simulink model "hx"  (R2021a)
settings: Solver=ode1  StartTime=0.0  StopTime=120  FixedStep=0.1  RelTol=1e-3
InitFcn:
  | hx_parameters
values from neighbouring files (symbols this model uses):
  A = 380    [hx_parameters.m]
  cp1 = 4190    [hx_parameters.m]
  cp2 = 4190    [hx_parameters.m]
  h = 6800    [hx_parameters.m]
  m1 = 400    [hx_parameters.m]
  m2 = 400    [hx_parameters.m]
  T1_ini = 68    [hx_parameters.m]
  T2_ini = 91    [hx_parameters.m]
settings Model: Creator=Mikael  LastModifiedBy=Mikael

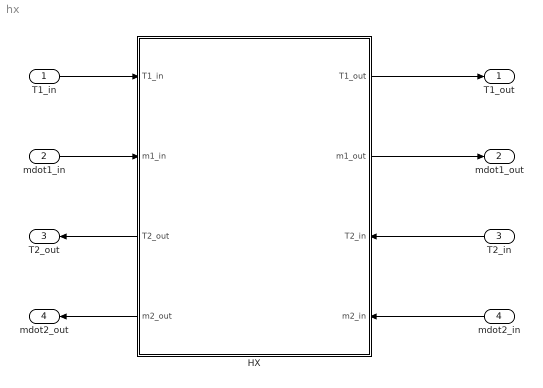
== system hx ==
  T1_in : Inport
  mdot1_in : Inport  Port=2
  T2_in : Inport  Port=3
  mdot2_in : Inport  Port=4
  HX : Subsystem
      settings: PortSchema="{\"entries\":[{\"content\":{\"sides\":[{\"content\":{\"connectorIds\":[\"In1\",\"In2\",\"Out3\",\"Out4\"]},\"type\":\"ConnectorPlacement.EquallySpacedRectSide\",\"uuid\":\"b608803e-13f5-49cd-ab3a-92503d47ac52\"},{\"content\":{\"connectorIds\":[\"Out1\",\"Out2\",\"In3\",\"In4\"],\"side\":\"RIGHT\"},\"type\":\"ConnectorPlacement.EquallySpacedRectSide\",\"uuid\":\"cb859c45-d915-447d-9a89-62abad3e0c6f\"},{\"content\":{\"connectorIds\":[],\"side\":\"TOP\"},\"type\":\"ConnectorPlacement.EquallySpacedRectSide\",\"uuid\":\"d365d95d-a075-458d-ace5-a17a7cf71809\"}]},\"type\":\"ConnectorPlacement.EquallySpacedConnector\",\"uuid\":\"ca673d01-47a6-46be-9ba4-be473b696b68\"}],\"packageUris\":[\"http://schema.mathworks.com/mf0/Connector/R2020b\"],\"version\":\"1.0\"}"
  T1_out : Outport
  mdot1_out : Outport  Port=2
  T2_out : Outport  Port=3
  mdot2_out : Outport  Port=4
  wires:
  T1_in/1 -> HX/1(T1_in)
  mdot1_in/1 -> HX/2(m1_in)
  T2_in/1 -> HX/3(T2_in)
  mdot2_in/1 -> HX/4(m2_in)
  HX/1(T1_out) -> T1_out/1
  HX/2(m1_out) -> mdot1_out/1
  HX/3(T2_out) -> T2_out/1
  HX/4(m2_out) -> mdot2_out/1

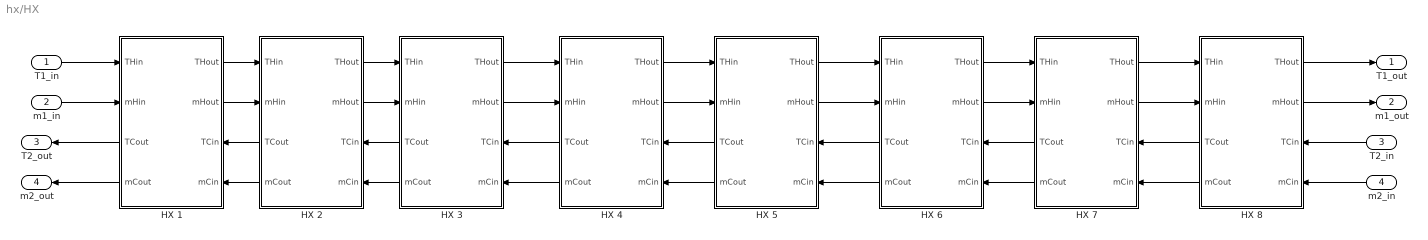
== system hx/HX ==
  T1_in : Inport
  m1_in : Inport  Port=2
  T2_in : Inport  Port=3
  m2_in : Inport  Port=4
  HX 1 : Subsystem
      settings: PortSchema="{\"entries\":[{\"content\":{\"sides\":[{\"content\":{\"connectorIds\":[\"In1\",\"In2\",\"Out3\",\"Out4\"]},\"type\":\"ConnectorPlacement.EquallySpacedRectSide\",\"uuid\":\"b608803e-13f5-49cd-ab3a-92503d47ac52\"},{\"content\":{\"connectorIds\":[\"Out1\",\"Out2\",\"In3\",\"In4\"],\"side\":\"RIGHT\"},\"type\":\"ConnectorPlacement.EquallySpacedRectSide\",\"uuid\":\"cb859c45-d915-447d-9a89-62abad3e0c6f\"},{\"content\":{\"connectorIds\":[],\"side\":\"TOP\"},\"type\":\"ConnectorPlacement.EquallySpacedRectSide\",\"uuid\":\"d365d95d-a075-458d-ace5-a17a7cf71809\"}]},\"type\":\"ConnectorPlacement.EquallySpacedConnector\",\"uuid\":\"ca673d01-47a6-46be-9ba4-be473b696b68\"}],\"packageUris\":[\"http://schema.mathworks.com/mf0/Connector/R2020b\"],\"version\":\"1.0\"}"
  HX 2 : Subsystem
      settings: PortSchema="{\"entries\":[{\"content\":{\"sides\":[{\"content\":{\"connectorIds\":[\"In1\",\"In2\",\"Out3\",\"Out4\"]},\"type\":\"ConnectorPlacement.EquallySpacedRectSide\",\"uuid\":\"b608803e-13f5-49cd-ab3a-92503d47ac52\"},{\"content\":{\"connectorIds\":[\"Out1\",\"Out2\",\"In3\",\"In4\"],\"side\":\"RIGHT\"},\"type\":\"ConnectorPlacement.EquallySpacedRectSide\",\"uuid\":\"cb859c45-d915-447d-9a89-62abad3e0c6f\"},{\"content\":{\"connectorIds\":[],\"side\":\"TOP\"},\"type\":\"ConnectorPlacement.EquallySpacedRectSide\",\"uuid\":\"d365d95d-a075-458d-ace5-a17a7cf71809\"}]},\"type\":\"ConnectorPlacement.EquallySpacedConnector\",\"uuid\":\"ca673d01-47a6-46be-9ba4-be473b696b68\"}],\"packageUris\":[\"http://schema.mathworks.com/mf0/Connector/R2020b\"],\"version\":\"1.0\"}"
  HX 3 : Subsystem
      settings: PortSchema="{\"entries\":[{\"content\":{\"sides\":[{\"content\":{\"connectorIds\":[\"In1\",\"In2\",\"Out3\",\"Out4\"]},\"type\":\"ConnectorPlacement.EquallySpacedRectSide\",\"uuid\":\"b608803e-13f5-49cd-ab3a-92503d47ac52\"},{\"content\":{\"connectorIds\":[\"Out1\",\"Out2\",\"In3\",\"In4\"],\"side\":\"RIGHT\"},\"type\":\"ConnectorPlacement.EquallySpacedRectSide\",\"uuid\":\"cb859c45-d915-447d-9a89-62abad3e0c6f\"},{\"content\":{\"connectorIds\":[],\"side\":\"TOP\"},\"type\":\"ConnectorPlacement.EquallySpacedRectSide\",\"uuid\":\"d365d95d-a075-458d-ace5-a17a7cf71809\"}]},\"type\":\"ConnectorPlacement.EquallySpacedConnector\",\"uuid\":\"ca673d01-47a6-46be-9ba4-be473b696b68\"}],\"packageUris\":[\"http://schema.mathworks.com/mf0/Connector/R2020b\"],\"version\":\"1.0\"}"
  HX 4 : Subsystem
      settings: PortSchema="{\"entries\":[{\"content\":{\"sides\":[{\"content\":{\"connectorIds\":[\"In1\",\"In2\",\"Out3\",\"Out4\"]},\"type\":\"ConnectorPlacement.EquallySpacedRectSide\",\"uuid\":\"b608803e-13f5-49cd-ab3a-92503d47ac52\"},{\"content\":{\"connectorIds\":[\"Out1\",\"Out2\",\"In3\",\"In4\"],\"side\":\"RIGHT\"},\"type\":\"ConnectorPlacement.EquallySpacedRectSide\",\"uuid\":\"cb859c45-d915-447d-9a89-62abad3e0c6f\"},{\"content\":{\"connectorIds\":[],\"side\":\"TOP\"},\"type\":\"ConnectorPlacement.EquallySpacedRectSide\",\"uuid\":\"d365d95d-a075-458d-ace5-a17a7cf71809\"}]},\"type\":\"ConnectorPlacement.EquallySpacedConnector\",\"uuid\":\"ca673d01-47a6-46be-9ba4-be473b696b68\"}],\"packageUris\":[\"http://schema.mathworks.com/mf0/Connector/R2020b\"],\"version\":\"1.0\"}"
  HX 5 : Subsystem
      settings: PortSchema="{\"entries\":[{\"content\":{\"sides\":[{\"content\":{\"connectorIds\":[\"In1\",\"In2\",\"Out3\",\"Out4\"]},\"type\":\"ConnectorPlacement.EquallySpacedRectSide\",\"uuid\":\"b608803e-13f5-49cd-ab3a-92503d47ac52\"},{\"content\":{\"connectorIds\":[\"Out1\",\"Out2\",\"In3\",\"In4\"],\"side\":\"RIGHT\"},\"type\":\"ConnectorPlacement.EquallySpacedRectSide\",\"uuid\":\"cb859c45-d915-447d-9a89-62abad3e0c6f\"},{\"content\":{\"connectorIds\":[],\"side\":\"TOP\"},\"type\":\"ConnectorPlacement.EquallySpacedRectSide\",\"uuid\":\"d365d95d-a075-458d-ace5-a17a7cf71809\"}]},\"type\":\"ConnectorPlacement.EquallySpacedConnector\",\"uuid\":\"ca673d01-47a6-46be-9ba4-be473b696b68\"}],\"packageUris\":[\"http://schema.mathworks.com/mf0/Connector/R2020b\"],\"version\":\"1.0\"}"
  HX 6 : Subsystem
      settings: PortSchema="{\"entries\":[{\"content\":{\"sides\":[{\"content\":{\"connectorIds\":[\"In1\",\"In2\",\"Out3\",\"Out4\"]},\"type\":\"ConnectorPlacement.EquallySpacedRectSide\",\"uuid\":\"b608803e-13f5-49cd-ab3a-92503d47ac52\"},{\"content\":{\"connectorIds\":[\"Out1\",\"Out2\",\"In3\",\"In4\"],\"side\":\"RIGHT\"},\"type\":\"ConnectorPlacement.EquallySpacedRectSide\",\"uuid\":\"cb859c45-d915-447d-9a89-62abad3e0c6f\"},{\"content\":{\"connectorIds\":[],\"side\":\"TOP\"},\"type\":\"ConnectorPlacement.EquallySpacedRectSide\",\"uuid\":\"d365d95d-a075-458d-ace5-a17a7cf71809\"}]},\"type\":\"ConnectorPlacement.EquallySpacedConnector\",\"uuid\":\"ca673d01-47a6-46be-9ba4-be473b696b68\"}],\"packageUris\":[\"http://schema.mathworks.com/mf0/Connector/R2020b\"],\"version\":\"1.0\"}"
  HX 7 : Subsystem
      settings: PortSchema="{\"entries\":[{\"content\":{\"sides\":[{\"content\":{\"connectorIds\":[\"In1\",\"In2\",\"Out3\",\"Out4\"]},\"type\":\"ConnectorPlacement.EquallySpacedRectSide\",\"uuid\":\"b608803e-13f5-49cd-ab3a-92503d47ac52\"},{\"content\":{\"connectorIds\":[\"Out1\",\"Out2\",\"In3\",\"In4\"],\"side\":\"RIGHT\"},\"type\":\"ConnectorPlacement.EquallySpacedRectSide\",\"uuid\":\"cb859c45-d915-447d-9a89-62abad3e0c6f\"},{\"content\":{\"connectorIds\":[],\"side\":\"TOP\"},\"type\":\"ConnectorPlacement.EquallySpacedRectSide\",\"uuid\":\"d365d95d-a075-458d-ace5-a17a7cf71809\"}]},\"type\":\"ConnectorPlacement.EquallySpacedConnector\",\"uuid\":\"ca673d01-47a6-46be-9ba4-be473b696b68\"}],\"packageUris\":[\"http://schema.mathworks.com/mf0/Connector/R2020b\"],\"version\":\"1.0\"}"
  HX 8 : Subsystem
      settings: PortSchema="{\"entries\":[{\"content\":{\"sides\":[{\"content\":{\"connectorIds\":[\"In1\",\"In2\",\"Out3\",\"Out4\"]},\"type\":\"ConnectorPlacement.EquallySpacedRectSide\",\"uuid\":\"b608803e-13f5-49cd-ab3a-92503d47ac52\"},{\"content\":{\"connectorIds\":[\"Out1\",\"Out2\",\"In3\",\"In4\"],\"side\":\"RIGHT\"},\"type\":\"ConnectorPlacement.EquallySpacedRectSide\",\"uuid\":\"cb859c45-d915-447d-9a89-62abad3e0c6f\"},{\"content\":{\"connectorIds\":[],\"side\":\"TOP\"},\"type\":\"ConnectorPlacement.EquallySpacedRectSide\",\"uuid\":\"d365d95d-a075-458d-ace5-a17a7cf71809\"}]},\"type\":\"ConnectorPlacement.EquallySpacedConnector\",\"uuid\":\"ca673d01-47a6-46be-9ba4-be473b696b68\"}],\"packageUris\":[\"http://schema.mathworks.com/mf0/Connector/R2020b\"],\"version\":\"1.0\"}"
  T1_out : Outport
  m1_out : Outport  Port=2
  T2_out : Outport  Port=3
  m2_out : Outport  Port=4
  wires:
  HX 2/3(TCout) -> HX 1/3(TCin)
  HX 4/1(THout) -> HX 5/1(THin)
  HX 4/2(mHout) -> HX 5/2(mHin)
  HX 1/1(THout) -> HX 2/1(THin)
  HX 5/3(TCout) -> HX 4/3(TCin)
  m1_in/1 -> HX 1/2(mHin)
  HX 2/1(THout) -> HX 3/1(THin)
  HX 1/2(mHout) -> HX 2/2(mHin)
  HX 5/4(mCout) -> HX 4/4(mCin)
  HX 2/4(mCout) -> HX 1/4(mCin)
  HX 5/2(mHout) -> HX 6/2(mHin)
  HX 7/4(mCout) -> HX 6/4(mCin)
  HX 7/3(TCout) -> HX 6/3(TCin)
  HX 3/2(mHout) -> HX 4/2(mHin)
  HX 6/2(mHout) -> HX 7/2(mHin)
  HX 8/2(mHout) -> m1_out/1
  HX 6/1(THout) -> HX 7/1(THin)
  HX 2/2(mHout) -> HX 3/2(mHin)
  HX 3/4(mCout) -> HX 2/4(mCin)
  T2_in/1 -> HX 8/3(TCin)
  HX 3/3(TCout) -> HX 2/3(TCin)
  T1_in/1 -> HX 1/1(THin)
  HX 5/1(THout) -> HX 6/1(THin)
  HX 3/1(THout) -> HX 4/1(THin)
  HX 4/3(TCout) -> HX 3/3(TCin)
  HX 6/3(TCout) -> HX 5/3(TCin)
  HX 4/4(mCout) -> HX 3/4(mCin)
  HX 7/1(THout) -> HX 8/1(THin)
  HX 8/3(TCout) -> HX 7/3(TCin)
  HX 7/2(mHout) -> HX 8/2(mHin)
  HX 8/4(mCout) -> HX 7/4(mCin)
  HX 1/3(TCout) -> T2_out/1
  HX 6/4(mCout) -> HX 5/4(mCin)
  HX 8/1(THout) -> T1_out/1
  m2_in/1 -> HX 8/4(mCin)
  HX 1/4(mCout) -> m2_out/1

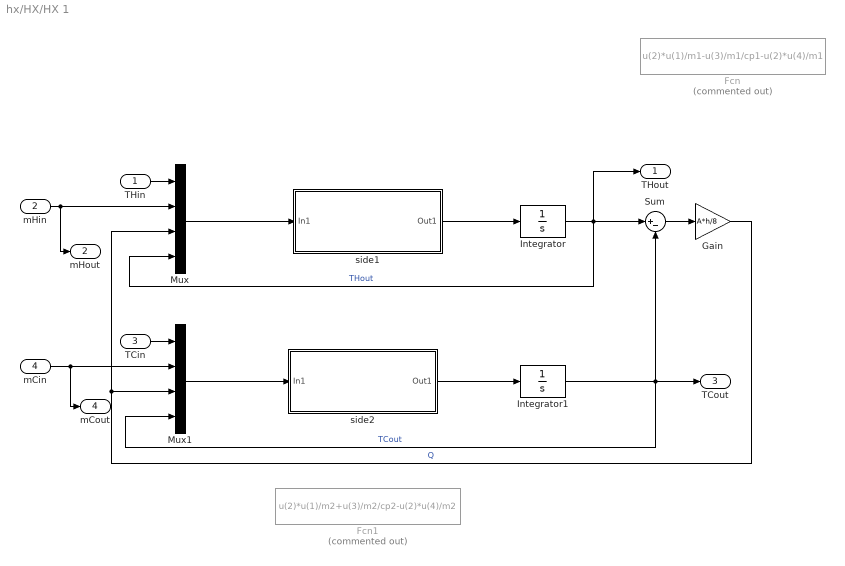
== system hx/HX/HX 1 ==
  THin : Inport
  mHin : Inport  Port=2
  TCin : Inport  Port=3
  mCin : Inport  Port=4
  Fcn : Fcn  Commented=on  Expr=u(2)*u(1)/m1-u(3)/m1/cp1-u(2)*u(4)/m1
  Fcn1 : Fcn  Commented=on  Expr=u(2)*u(1)/m2+u(3)/m2/cp2-u(2)*u(4)/m2
  Gain : Gain  Gain=A*h/8
  Integrator : Integrator  InitialCondition=T1_ini
  Integrator1 : Integrator  InitialCondition=T2_ini
  Mux : Mux
  Mux1 : Mux
  Sum : Sum  Inputs=|+-
  side1 : Subsystem
  side2 : Subsystem
  THout : Outport  VectorParamsAs1DForOutWhenUnconnected=off
  mHout : Outport  Port=2  VectorParamsAs1DForOutWhenUnconnected=off
  TCout : Outport  Port=3  VectorParamsAs1DForOutWhenUnconnected=off
  mCout : Outport  Port=4  VectorParamsAs1DForOutWhenUnconnected=off
  wires:
  Integrator/1 -> THout/1, Sum/1, Mux/4  "THout"
  Sum/1 -> Gain/1
  Mux1/1 -> side2/1(In1)
  side2/1(Out1) -> Integrator1/1
  Integrator1/1 -> Sum/2, TCout/1, Mux1/4  "TCout"
  mCin/1 -> Mux1/2, mCout/1
  TCin/1 -> Mux1/1
  THin/1 -> Mux/1
  Gain/1 -> Mux1/3, Mux/3  "Q"
  mHin/1 -> Mux/2, mHout/1
  Mux/1 -> side1/1(In1)
  side1/1(Out1) -> Integrator/1

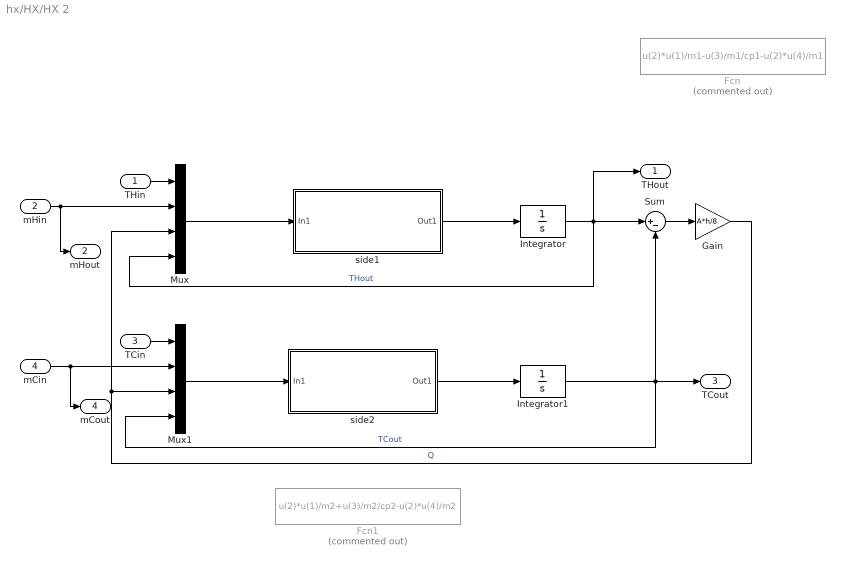
== system hx/HX/HX 2 ==
  THin : Inport
  mHin : Inport  Port=2
  TCin : Inport  Port=3
  mCin : Inport  Port=4
  Fcn : Fcn  Commented=on  Expr=u(2)*u(1)/m1-u(3)/m1/cp1-u(2)*u(4)/m1
  Fcn1 : Fcn  Commented=on  Expr=u(2)*u(1)/m2+u(3)/m2/cp2-u(2)*u(4)/m2
  Gain : Gain  Gain=A*h/8
  Integrator : Integrator  InitialCondition=T1_ini
  Integrator1 : Integrator  InitialCondition=T2_ini
  Mux : Mux
  Mux1 : Mux
  Sum : Sum  Inputs=|+-
  side1 : Subsystem
  side2 : Subsystem
  THout : Outport  VectorParamsAs1DForOutWhenUnconnected=off
  mHout : Outport  Port=2  VectorParamsAs1DForOutWhenUnconnected=off
  TCout : Outport  Port=3  VectorParamsAs1DForOutWhenUnconnected=off
  mCout : Outport  Port=4  VectorParamsAs1DForOutWhenUnconnected=off
  wires:
  side1/1(Out1) -> Integrator/1
  Mux/1 -> side1/1(In1)
  mHin/1 -> mHout/1, Mux/2
  Gain/1 -> Mux/3, Mux1/3  "Q"
  THin/1 -> Mux/1
  TCin/1 -> Mux1/1
  mCin/1 -> mCout/1, Mux1/2
  Integrator1/1 -> Mux1/4, TCout/1, Sum/2  "TCout"
  side2/1(Out1) -> Integrator1/1
  Mux1/1 -> side2/1(In1)
  Sum/1 -> Gain/1
  Integrator/1 -> Mux/4, Sum/1, THout/1  "THout"

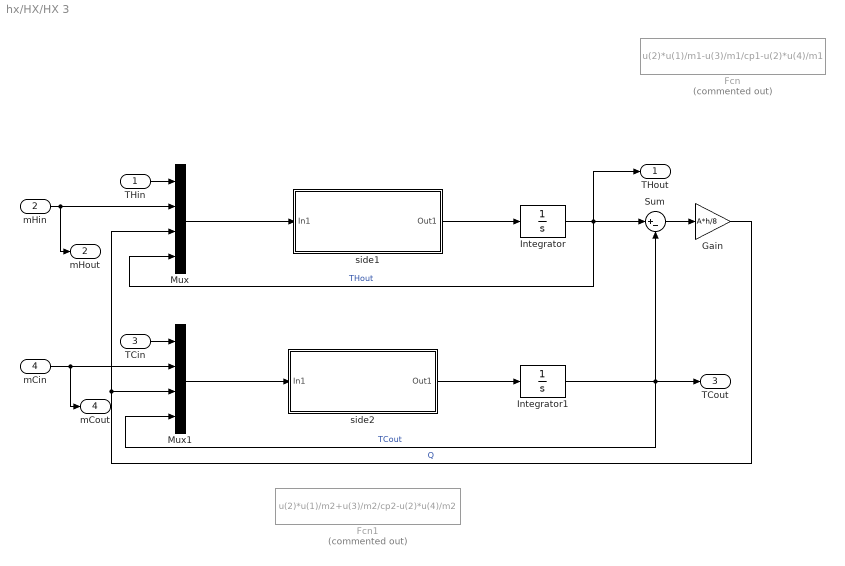
== system hx/HX/HX 3 ==
  THin : Inport
  mHin : Inport  Port=2
  TCin : Inport  Port=3
  mCin : Inport  Port=4
  Fcn : Fcn  Commented=on  Expr=u(2)*u(1)/m1-u(3)/m1/cp1-u(2)*u(4)/m1
  Fcn1 : Fcn  Commented=on  Expr=u(2)*u(1)/m2+u(3)/m2/cp2-u(2)*u(4)/m2
  Gain : Gain  Gain=A*h/8
  Integrator : Integrator  InitialCondition=T1_ini
  Integrator1 : Integrator  InitialCondition=T2_ini
  Mux : Mux
  Mux1 : Mux
  Sum : Sum  Inputs=|+-
  side1 : Subsystem
  side2 : Subsystem
  THout : Outport  VectorParamsAs1DForOutWhenUnconnected=off
  mHout : Outport  Port=2  VectorParamsAs1DForOutWhenUnconnected=off
  TCout : Outport  Port=3  VectorParamsAs1DForOutWhenUnconnected=off
  mCout : Outport  Port=4  VectorParamsAs1DForOutWhenUnconnected=off
  wires:
  Integrator/1 -> THout/1, Sum/1, Mux/4  "THout"
  Sum/1 -> Gain/1
  Mux1/1 -> side2/1(In1)
  side2/1(Out1) -> Integrator1/1
  Integrator1/1 -> Sum/2, TCout/1, Mux1/4  "TCout"
  mCin/1 -> Mux1/2, mCout/1
  TCin/1 -> Mux1/1
  THin/1 -> Mux/1
  Gain/1 -> Mux1/3, Mux/3  "Q"
  mHin/1 -> Mux/2, mHout/1
  Mux/1 -> side1/1(In1)
  side1/1(Out1) -> Integrator/1

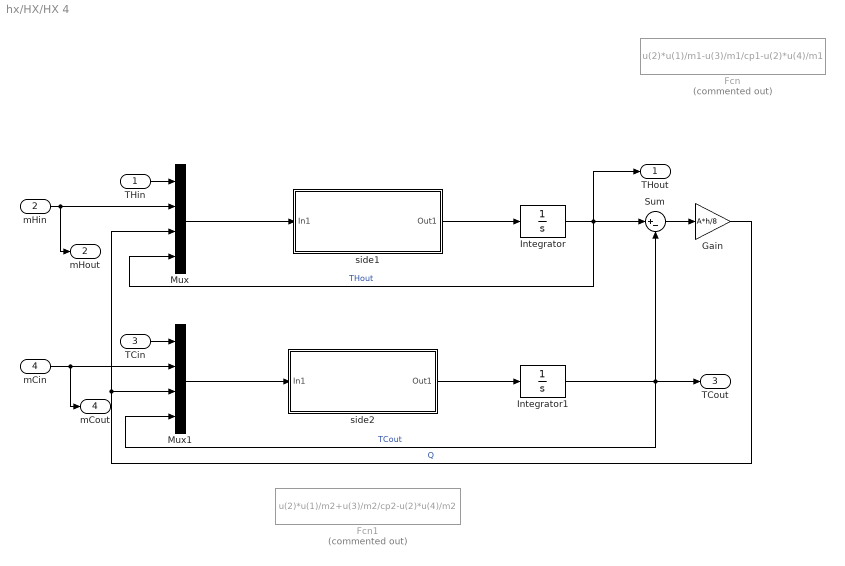
== system hx/HX/HX 4 ==
  THin : Inport
  mHin : Inport  Port=2
  TCin : Inport  Port=3
  mCin : Inport  Port=4
  Fcn : Fcn  Commented=on  Expr=u(2)*u(1)/m1-u(3)/m1/cp1-u(2)*u(4)/m1
  Fcn1 : Fcn  Commented=on  Expr=u(2)*u(1)/m2+u(3)/m2/cp2-u(2)*u(4)/m2
  Gain : Gain  Gain=A*h/8
  Integrator : Integrator  InitialCondition=T1_ini
  Integrator1 : Integrator  InitialCondition=T2_ini
  Mux : Mux
  Mux1 : Mux
  Sum : Sum  Inputs=|+-
  side1 : Subsystem
  side2 : Subsystem
  THout : Outport  VectorParamsAs1DForOutWhenUnconnected=off
  mHout : Outport  Port=2  VectorParamsAs1DForOutWhenUnconnected=off
  TCout : Outport  Port=3  VectorParamsAs1DForOutWhenUnconnected=off
  mCout : Outport  Port=4  VectorParamsAs1DForOutWhenUnconnected=off
  wires:
  side1/1(Out1) -> Integrator/1
  Mux/1 -> side1/1(In1)
  mHin/1 -> mHout/1, Mux/2
  Gain/1 -> Mux/3, Mux1/3  "Q"
  THin/1 -> Mux/1
  TCin/1 -> Mux1/1
  mCin/1 -> mCout/1, Mux1/2
  Integrator1/1 -> Mux1/4, TCout/1, Sum/2  "TCout"
  side2/1(Out1) -> Integrator1/1
  Mux1/1 -> side2/1(In1)
  Sum/1 -> Gain/1
  Integrator/1 -> Mux/4, Sum/1, THout/1  "THout"

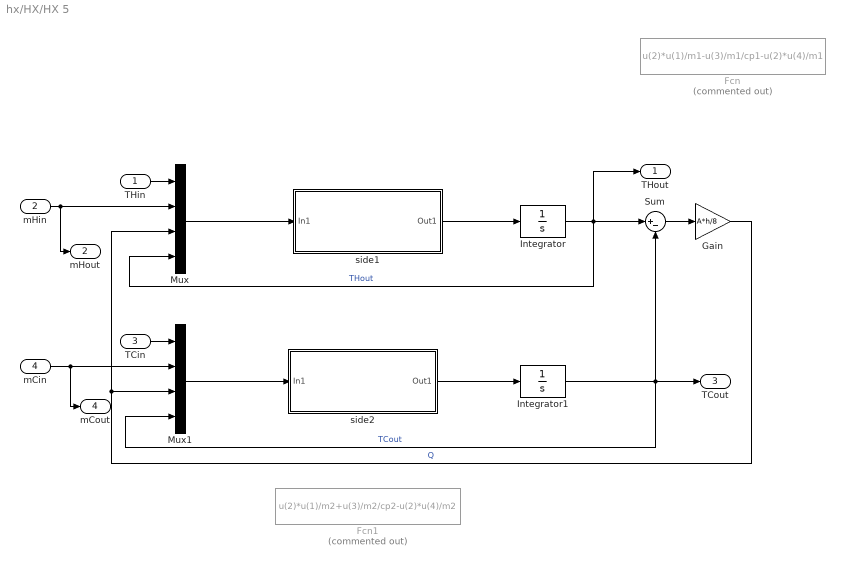
== system hx/HX/HX 5 ==
  THin : Inport
  mHin : Inport  Port=2
  TCin : Inport  Port=3
  mCin : Inport  Port=4
  Fcn : Fcn  Commented=on  Expr=u(2)*u(1)/m1-u(3)/m1/cp1-u(2)*u(4)/m1
  Fcn1 : Fcn  Commented=on  Expr=u(2)*u(1)/m2+u(3)/m2/cp2-u(2)*u(4)/m2
  Gain : Gain  Gain=A*h/8
  Integrator : Integrator  InitialCondition=T1_ini
  Integrator1 : Integrator  InitialCondition=T2_ini
  Mux : Mux
  Mux1 : Mux
  Sum : Sum  Inputs=|+-
  side1 : Subsystem
  side2 : Subsystem
  THout : Outport  VectorParamsAs1DForOutWhenUnconnected=off
  mHout : Outport  Port=2  VectorParamsAs1DForOutWhenUnconnected=off
  TCout : Outport  Port=3  VectorParamsAs1DForOutWhenUnconnected=off
  mCout : Outport  Port=4  VectorParamsAs1DForOutWhenUnconnected=off
  wires:
  Integrator/1 -> THout/1, Sum/1, Mux/4  "THout"
  Sum/1 -> Gain/1
  Mux1/1 -> side2/1(In1)
  side2/1(Out1) -> Integrator1/1
  Integrator1/1 -> Sum/2, TCout/1, Mux1/4  "TCout"
  mCin/1 -> Mux1/2, mCout/1
  TCin/1 -> Mux1/1
  THin/1 -> Mux/1
  Gain/1 -> Mux1/3, Mux/3  "Q"
  mHin/1 -> Mux/2, mHout/1
  Mux/1 -> side1/1(In1)
  side1/1(Out1) -> Integrator/1

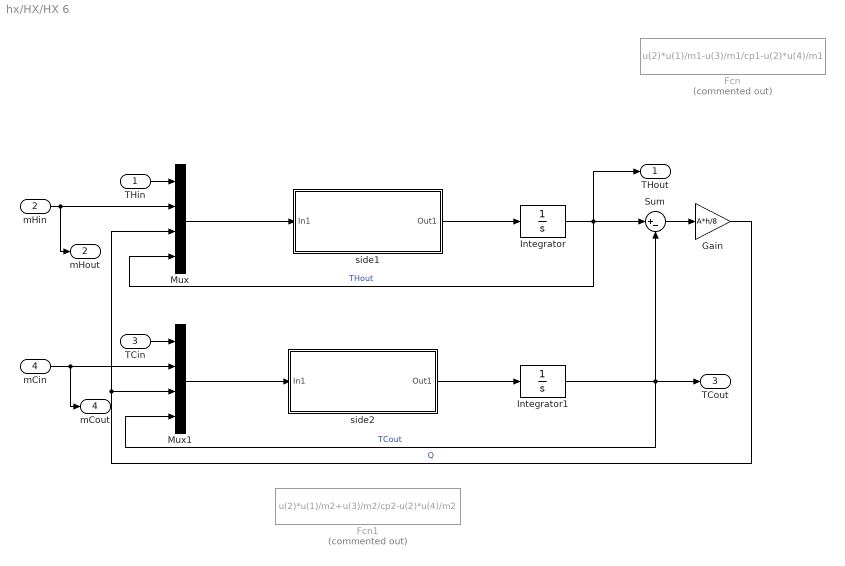
== system hx/HX/HX 6 ==
  THin : Inport
  mHin : Inport  Port=2
  TCin : Inport  Port=3
  mCin : Inport  Port=4
  Fcn : Fcn  Commented=on  Expr=u(2)*u(1)/m1-u(3)/m1/cp1-u(2)*u(4)/m1
  Fcn1 : Fcn  Commented=on  Expr=u(2)*u(1)/m2+u(3)/m2/cp2-u(2)*u(4)/m2
  Gain : Gain  Gain=A*h/8
  Integrator : Integrator  InitialCondition=T1_ini
  Integrator1 : Integrator  InitialCondition=T2_ini
  Mux : Mux
  Mux1 : Mux
  Sum : Sum  Inputs=|+-
  side1 : Subsystem
  side2 : Subsystem
  THout : Outport  VectorParamsAs1DForOutWhenUnconnected=off
  mHout : Outport  Port=2  VectorParamsAs1DForOutWhenUnconnected=off
  TCout : Outport  Port=3  VectorParamsAs1DForOutWhenUnconnected=off
  mCout : Outport  Port=4  VectorParamsAs1DForOutWhenUnconnected=off
  wires:
  side1/1(Out1) -> Integrator/1
  Mux/1 -> side1/1(In1)
  mHin/1 -> mHout/1, Mux/2
  Gain/1 -> Mux/3, Mux1/3  "Q"
  THin/1 -> Mux/1
  TCin/1 -> Mux1/1
  mCin/1 -> mCout/1, Mux1/2
  Integrator1/1 -> Mux1/4, TCout/1, Sum/2  "TCout"
  side2/1(Out1) -> Integrator1/1
  Mux1/1 -> side2/1(In1)
  Sum/1 -> Gain/1
  Integrator/1 -> Mux/4, Sum/1, THout/1  "THout"

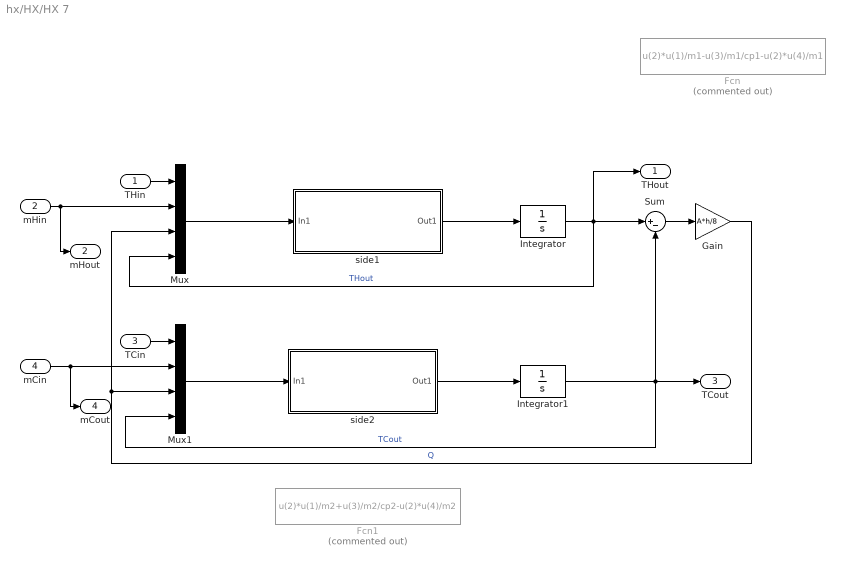
== system hx/HX/HX 7 ==
  THin : Inport
  mHin : Inport  Port=2
  TCin : Inport  Port=3
  mCin : Inport  Port=4
  Fcn : Fcn  Commented=on  Expr=u(2)*u(1)/m1-u(3)/m1/cp1-u(2)*u(4)/m1
  Fcn1 : Fcn  Commented=on  Expr=u(2)*u(1)/m2+u(3)/m2/cp2-u(2)*u(4)/m2
  Gain : Gain  Gain=A*h/8
  Integrator : Integrator  InitialCondition=T1_ini
  Integrator1 : Integrator  InitialCondition=T2_ini
  Mux : Mux
  Mux1 : Mux
  Sum : Sum  Inputs=|+-
  side1 : Subsystem
  side2 : Subsystem
  THout : Outport  VectorParamsAs1DForOutWhenUnconnected=off
  mHout : Outport  Port=2  VectorParamsAs1DForOutWhenUnconnected=off
  TCout : Outport  Port=3  VectorParamsAs1DForOutWhenUnconnected=off
  mCout : Outport  Port=4  VectorParamsAs1DForOutWhenUnconnected=off
  wires:
  Integrator/1 -> THout/1, Sum/1, Mux/4  "THout"
  Sum/1 -> Gain/1
  Mux1/1 -> side2/1(In1)
  side2/1(Out1) -> Integrator1/1
  Integrator1/1 -> Sum/2, TCout/1, Mux1/4  "TCout"
  mCin/1 -> Mux1/2, mCout/1
  TCin/1 -> Mux1/1
  THin/1 -> Mux/1
  Gain/1 -> Mux1/3, Mux/3  "Q"
  mHin/1 -> Mux/2, mHout/1
  Mux/1 -> side1/1(In1)
  side1/1(Out1) -> Integrator/1

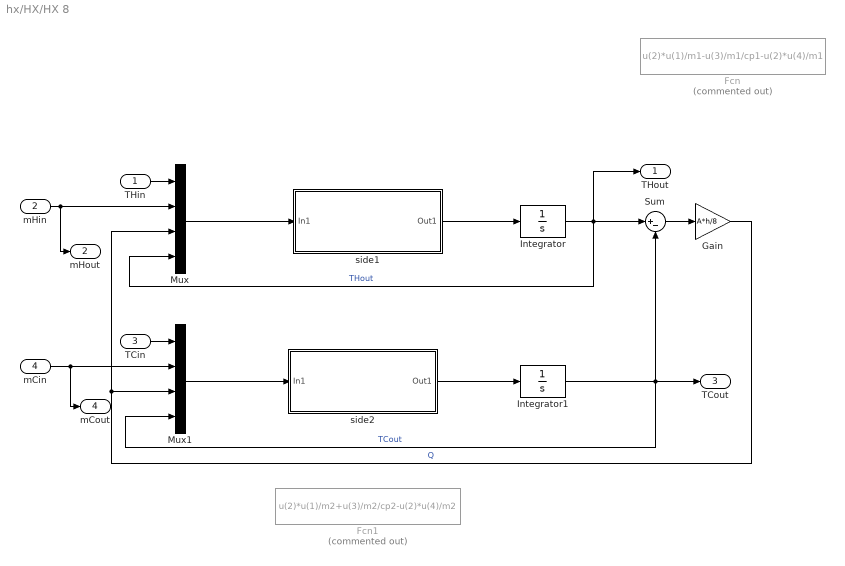
== system hx/HX/HX 8 ==
  THin : Inport
  mHin : Inport  Port=2
  TCin : Inport  Port=3
  mCin : Inport  Port=4
  Fcn : Fcn  Commented=on  Expr=u(2)*u(1)/m1-u(3)/m1/cp1-u(2)*u(4)/m1
  Fcn1 : Fcn  Commented=on  Expr=u(2)*u(1)/m2+u(3)/m2/cp2-u(2)*u(4)/m2
  Gain : Gain  Gain=A*h/8
  Integrator : Integrator  InitialCondition=T1_ini
  Integrator1 : Integrator  InitialCondition=T2_ini
  Mux : Mux
  Mux1 : Mux
  Sum : Sum  Inputs=|+-
  side1 : Subsystem
  side2 : Subsystem
  THout : Outport  VectorParamsAs1DForOutWhenUnconnected=off
  mHout : Outport  Port=2  VectorParamsAs1DForOutWhenUnconnected=off
  TCout : Outport  Port=3  VectorParamsAs1DForOutWhenUnconnected=off
  mCout : Outport  Port=4  VectorParamsAs1DForOutWhenUnconnected=off
  wires:
  side1/1(Out1) -> Integrator/1
  Mux/1 -> side1/1(In1)
  mHin/1 -> mHout/1, Mux/2
  Gain/1 -> Mux/3, Mux1/3  "Q"
  THin/1 -> Mux/1
  TCin/1 -> Mux1/1
  mCin/1 -> mCout/1, Mux1/2
  Integrator1/1 -> Mux1/4, TCout/1, Sum/2  "TCout"
  side2/1(Out1) -> Integrator1/1
  Mux1/1 -> side2/1(In1)
  Sum/1 -> Gain/1
  Integrator/1 -> Mux/4, Sum/1, THout/1  "THout"

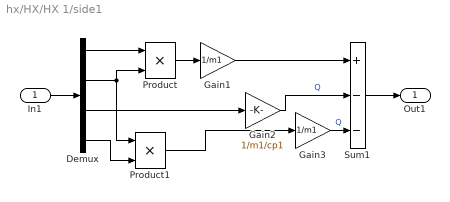
== system hx/HX/HX 1/side1 ==
  In1 : Inport
  Demux : Demux
  Gain1 : Gain  Gain=1/m1
  Gain2 : Gain  Gain=1/m1/cp1
  Gain3 : Gain  Gain=1/m1
  Product : Product
  Product1 : Product
  Sum1 : Sum  Inputs=+--
  Out1 : Outport
  wires:
  Demux/4 -> Product1/2
  Demux/3 -> Gain2/1
  Product1/1 -> Gain3/1
  Gain2/1 -> Sum1/2  "Q"
  Demux/2 -> Product/2, Product1/1
  Demux/1 -> Product/1
  Gain3/1 -> Sum1/3  "Q"
  Product/1 -> Gain1/1
  Gain1/1 -> Sum1/1
  Sum1/1 -> Out1/1
  In1/1 -> Demux/1

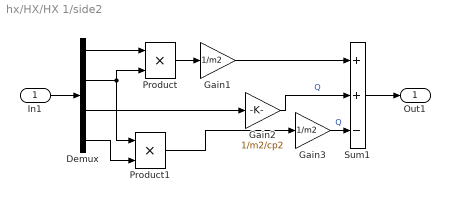
== system hx/HX/HX 1/side2 ==
  In1 : Inport
  Demux : Demux
  Gain1 : Gain  Gain=1/m2
  Gain2 : Gain  Gain=1/m2/cp2
  Gain3 : Gain  Gain=1/m2
  Product : Product
  Product1 : Product
  Sum1 : Sum  Inputs=++-
  Out1 : Outport
  wires:
  In1/1 -> Demux/1
  Sum1/1 -> Out1/1
  Gain1/1 -> Sum1/1
  Product/1 -> Gain1/1
  Gain3/1 -> Sum1/3  "Q"
  Demux/1 -> Product/1
  Demux/2 -> Product1/1, Product/2
  Gain2/1 -> Sum1/2  "Q"
  Product1/1 -> Gain3/1
  Demux/3 -> Gain2/1
  Demux/4 -> Product1/2

== system hx/HX/HX 2/side1 ==
  In1 : Inport
  Demux : Demux
  Gain1 : Gain  Gain=1/m1
  Gain2 : Gain  Gain=1/m1/cp1
  Gain3 : Gain  Gain=1/m1
  Product : Product
  Product1 : Product
  Sum1 : Sum  Inputs=+--
  Out1 : Outport
  wires:
  In1/1 -> Demux/1
  Sum1/1 -> Out1/1
  Gain1/1 -> Sum1/1
  Product/1 -> Gain1/1
  Gain3/1 -> Sum1/3  "Q"
  Demux/1 -> Product/1
  Demux/2 -> Product1/1, Product/2
  Gain2/1 -> Sum1/2  "Q"
  Product1/1 -> Gain3/1
  Demux/3 -> Gain2/1
  Demux/4 -> Product1/2

== system hx/HX/HX 2/side2 ==
  In1 : Inport
  Demux : Demux
  Gain1 : Gain  Gain=1/m2
  Gain2 : Gain  Gain=1/m2/cp2
  Gain3 : Gain  Gain=1/m2
  Product : Product
  Product1 : Product
  Sum1 : Sum  Inputs=++-
  Out1 : Outport
  wires:
  Demux/4 -> Product1/2
  Demux/3 -> Gain2/1
  Product1/1 -> Gain3/1
  Gain2/1 -> Sum1/2  "Q"
  Demux/2 -> Product/2, Product1/1
  Demux/1 -> Product/1
  Gain3/1 -> Sum1/3  "Q"
  Product/1 -> Gain1/1
  Gain1/1 -> Sum1/1
  Sum1/1 -> Out1/1
  In1/1 -> Demux/1

== system hx/HX/HX 3/side1 ==
  In1 : Inport
  Demux : Demux
  Gain1 : Gain  Gain=1/m1
  Gain2 : Gain  Gain=1/m1/cp1
  Gain3 : Gain  Gain=1/m1
  Product : Product
  Product1 : Product
  Sum1 : Sum  Inputs=+--
  Out1 : Outport
  wires:
  Demux/4 -> Product1/2
  Demux/3 -> Gain2/1
  Product1/1 -> Gain3/1
  Gain2/1 -> Sum1/2  "Q"
  Demux/2 -> Product/2, Product1/1
  Demux/1 -> Product/1
  Gain3/1 -> Sum1/3  "Q"
  Product/1 -> Gain1/1
  Gain1/1 -> Sum1/1
  Sum1/1 -> Out1/1
  In1/1 -> Demux/1

== system hx/HX/HX 3/side2 ==
  In1 : Inport
  Demux : Demux
  Gain1 : Gain  Gain=1/m2
  Gain2 : Gain  Gain=1/m2/cp2
  Gain3 : Gain  Gain=1/m2
  Product : Product
  Product1 : Product
  Sum1 : Sum  Inputs=++-
  Out1 : Outport
  wires:
  In1/1 -> Demux/1
  Sum1/1 -> Out1/1
  Gain1/1 -> Sum1/1
  Product/1 -> Gain1/1
  Gain3/1 -> Sum1/3  "Q"
  Demux/1 -> Product/1
  Demux/2 -> Product1/1, Product/2
  Gain2/1 -> Sum1/2  "Q"
  Product1/1 -> Gain3/1
  Demux/3 -> Gain2/1
  Demux/4 -> Product1/2

== system hx/HX/HX 4/side1 ==
  In1 : Inport
  Demux : Demux
  Gain1 : Gain  Gain=1/m1
  Gain2 : Gain  Gain=1/m1/cp1
  Gain3 : Gain  Gain=1/m1
  Product : Product
  Product1 : Product
  Sum1 : Sum  Inputs=+--
  Out1 : Outport
  wires:
  In1/1 -> Demux/1
  Sum1/1 -> Out1/1
  Gain1/1 -> Sum1/1
  Product/1 -> Gain1/1
  Gain3/1 -> Sum1/3  "Q"
  Demux/1 -> Product/1
  Demux/2 -> Product1/1, Product/2
  Gain2/1 -> Sum1/2  "Q"
  Product1/1 -> Gain3/1
  Demux/3 -> Gain2/1
  Demux/4 -> Product1/2

== system hx/HX/HX 4/side2 ==
  In1 : Inport
  Demux : Demux
  Gain1 : Gain  Gain=1/m2
  Gain2 : Gain  Gain=1/m2/cp2
  Gain3 : Gain  Gain=1/m2
  Product : Product
  Product1 : Product
  Sum1 : Sum  Inputs=++-
  Out1 : Outport
  wires:
  Demux/4 -> Product1/2
  Demux/3 -> Gain2/1
  Product1/1 -> Gain3/1
  Gain2/1 -> Sum1/2  "Q"
  Demux/2 -> Product/2, Product1/1
  Demux/1 -> Product/1
  Gain3/1 -> Sum1/3  "Q"
  Product/1 -> Gain1/1
  Gain1/1 -> Sum1/1
  Sum1/1 -> Out1/1
  In1/1 -> Demux/1

== system hx/HX/HX 5/side1 ==
  In1 : Inport
  Demux : Demux
  Gain1 : Gain  Gain=1/m1
  Gain2 : Gain  Gain=1/m1/cp1
  Gain3 : Gain  Gain=1/m1
  Product : Product
  Product1 : Product
  Sum1 : Sum  Inputs=+--
  Out1 : Outport
  wires:
  Demux/4 -> Product1/2
  Demux/3 -> Gain2/1
  Product1/1 -> Gain3/1
  Gain2/1 -> Sum1/2  "Q"
  Demux/2 -> Product/2, Product1/1
  Demux/1 -> Product/1
  Gain3/1 -> Sum1/3  "Q"
  Product/1 -> Gain1/1
  Gain1/1 -> Sum1/1
  Sum1/1 -> Out1/1
  In1/1 -> Demux/1

== system hx/HX/HX 5/side2 ==
  In1 : Inport
  Demux : Demux
  Gain1 : Gain  Gain=1/m2
  Gain2 : Gain  Gain=1/m2/cp2
  Gain3 : Gain  Gain=1/m2
  Product : Product
  Product1 : Product
  Sum1 : Sum  Inputs=++-
  Out1 : Outport
  wires:
  In1/1 -> Demux/1
  Sum1/1 -> Out1/1
  Gain1/1 -> Sum1/1
  Product/1 -> Gain1/1
  Gain3/1 -> Sum1/3  "Q"
  Demux/1 -> Product/1
  Demux/2 -> Product1/1, Product/2
  Gain2/1 -> Sum1/2  "Q"
  Product1/1 -> Gain3/1
  Demux/3 -> Gain2/1
  Demux/4 -> Product1/2

== system hx/HX/HX 6/side1 ==
  In1 : Inport
  Demux : Demux
  Gain1 : Gain  Gain=1/m1
  Gain2 : Gain  Gain=1/m1/cp1
  Gain3 : Gain  Gain=1/m1
  Product : Product
  Product1 : Product
  Sum1 : Sum  Inputs=+--
  Out1 : Outport
  wires:
  In1/1 -> Demux/1
  Sum1/1 -> Out1/1
  Gain1/1 -> Sum1/1
  Product/1 -> Gain1/1
  Gain3/1 -> Sum1/3  "Q"
  Demux/1 -> Product/1
  Demux/2 -> Product1/1, Product/2
  Gain2/1 -> Sum1/2  "Q"
  Product1/1 -> Gain3/1
  Demux/3 -> Gain2/1
  Demux/4 -> Product1/2

== system hx/HX/HX 6/side2 ==
  In1 : Inport
  Demux : Demux
  Gain1 : Gain  Gain=1/m2
  Gain2 : Gain  Gain=1/m2/cp2
  Gain3 : Gain  Gain=1/m2
  Product : Product
  Product1 : Product
  Sum1 : Sum  Inputs=++-
  Out1 : Outport
  wires:
  Demux/4 -> Product1/2
  Demux/3 -> Gain2/1
  Product1/1 -> Gain3/1
  Gain2/1 -> Sum1/2  "Q"
  Demux/2 -> Product/2, Product1/1
  Demux/1 -> Product/1
  Gain3/1 -> Sum1/3  "Q"
  Product/1 -> Gain1/1
  Gain1/1 -> Sum1/1
  Sum1/1 -> Out1/1
  In1/1 -> Demux/1

== system hx/HX/HX 7/side1 ==
  In1 : Inport
  Demux : Demux
  Gain1 : Gain  Gain=1/m1
  Gain2 : Gain  Gain=1/m1/cp1
  Gain3 : Gain  Gain=1/m1
  Product : Product
  Product1 : Product
  Sum1 : Sum  Inputs=+--
  Out1 : Outport
  wires:
  Demux/4 -> Product1/2
  Demux/3 -> Gain2/1
  Product1/1 -> Gain3/1
  Gain2/1 -> Sum1/2  "Q"
  Demux/2 -> Product/2, Product1/1
  Demux/1 -> Product/1
  Gain3/1 -> Sum1/3  "Q"
  Product/1 -> Gain1/1
  Gain1/1 -> Sum1/1
  Sum1/1 -> Out1/1
  In1/1 -> Demux/1

== system hx/HX/HX 7/side2 ==
  In1 : Inport
  Demux : Demux
  Gain1 : Gain  Gain=1/m2
  Gain2 : Gain  Gain=1/m2/cp2
  Gain3 : Gain  Gain=1/m2
  Product : Product
  Product1 : Product
  Sum1 : Sum  Inputs=++-
  Out1 : Outport
  wires:
  In1/1 -> Demux/1
  Sum1/1 -> Out1/1
  Gain1/1 -> Sum1/1
  Product/1 -> Gain1/1
  Gain3/1 -> Sum1/3  "Q"
  Demux/1 -> Product/1
  Demux/2 -> Product1/1, Product/2
  Gain2/1 -> Sum1/2  "Q"
  Product1/1 -> Gain3/1
  Demux/3 -> Gain2/1
  Demux/4 -> Product1/2

== system hx/HX/HX 8/side1 ==
  In1 : Inport
  Demux : Demux
  Gain1 : Gain  Gain=1/m1
  Gain2 : Gain  Gain=1/m1/cp1
  Gain3 : Gain  Gain=1/m1
  Product : Product
  Product1 : Product
  Sum1 : Sum  Inputs=+--
  Out1 : Outport
  wires:
  In1/1 -> Demux/1
  Sum1/1 -> Out1/1
  Gain1/1 -> Sum1/1
  Product/1 -> Gain1/1
  Gain3/1 -> Sum1/3  "Q"
  Demux/1 -> Product/1
  Demux/2 -> Product1/1, Product/2
  Gain2/1 -> Sum1/2  "Q"
  Product1/1 -> Gain3/1
  Demux/3 -> Gain2/1
  Demux/4 -> Product1/2

== system hx/HX/HX 8/side2 ==
  In1 : Inport
  Demux : Demux
  Gain1 : Gain  Gain=1/m2
  Gain2 : Gain  Gain=1/m2/cp2
  Gain3 : Gain  Gain=1/m2
  Product : Product
  Product1 : Product
  Sum1 : Sum  Inputs=++-
  Out1 : Outport
  wires:
  Demux/4 -> Product1/2
  Demux/3 -> Gain2/1
  Product1/1 -> Gain3/1
  Gain2/1 -> Sum1/2  "Q"
  Demux/2 -> Product/2, Product1/1
  Demux/1 -> Product/1
  Gain3/1 -> Sum1/3  "Q"
  Product/1 -> Gain1/1
  Gain1/1 -> Sum1/1
  Sum1/1 -> Out1/1
  In1/1 -> Demux/1
